simulink model "osek_led"  (Simulink 6.0)
settings: Solver=FixedStepDiscrete  StartTime=0.0  StopTime=100.0  RelTol=1e-3
undefined symbols (not defined in the file or in its folder): D4, D5, green, red
libraries: simulink x2, osekdrivers x2
settings Model: Creator=jcarrick  LastModifiedBy=jcarrick  ProdHWDeviceType=Motorola PowerPC
settings SolverCC: PositivePriorityOrder=on
settings DataIOCC: SaveOutput=off  SaveTime=off  SignalLoggingName=sigsOut
settings OptimizationCC: InlineInvariantSignals=off  OptimizeModelRefInitCode=on  LifeSpan=1
settings DebuggingCC: CheckExecutionContextPreStartOutputMsg=on  CheckExecutionContextRuntimeOutputMsg=on  SolverPrmCheckMsg=none
settings HardwareCC: ProdEndianess=BigEndian  ProdHWDeviceType=Motorola PowerPC
settings RTWCC: SystemTargetFile=osekworks.tlc  GenCodeOnly=on  TemplateMakefile=osek_default_tmf  GenerateReport=on  ProcessScript=osekworks_make_rtw_hook  IncludeHyperlinkInReport=on  LaunchReport=on
settings CodeAppCC: IgnoreCustomStorageClasses=off
settings STFCustomTargetCC: TargetFcnLib=ansi_tfl_tmw.mat  GenFloatMathFcnCalls=ANSI_C  ModelReferenceCompliant=off  CombineOutputUpdateFcns=on  SuppressErrorStatus=on  ERTCustomFileBanners=on  PurelyIntegerCode=on  SystemTargetFile=proosek.tlc  ForcedBaseTarget=off
settings ERTTargetCC: TargetFcnLib=ansi_tfl_tmw.mat  GenFloatMathFcnCalls=ANSI_C  ModelReferenceCompliant=off  SuppressErrorStatus=on  PurelyIntegerCode=on  SupportContinuousTime=on  SupportNonInlinedSFcns=on  RootIOFormat=Individual Arguments  ERTCustomFileTemplate=osek_file_process.tlc  InitialValueSource=Model
settings CustomProperty: DataType=RTWOptions_EnumType__toolbox_rtw_targets_osek_osek_osekworks_bspName  Value=phycore555
settings EnumStrPairs: String=axiomcmd565
settings SFSimCC: SFSimApplyToAllLibs=on  SFSimBuildMode=Incremental

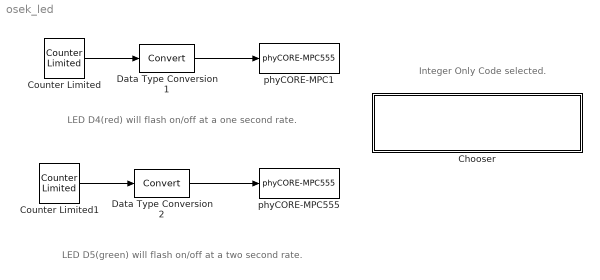
== system osek_led ==
  note: LED D4(red) will flash on/off at a one second rate.
  note: LED D5(green) will flash on/off at a two second rate.
  note: Integer Only Code selected.
  Chooser : Subsystem  LoadFcn=|  PropExecContextAcrossSSBoundary=on  mask{stf=osekworks.tlc}
      | x = osek.prefs.load('osek');                               
      | Implementation = lower(x.Implementation);                  
      | clear x;                                                   
      | switch Implementation                                      
      |  case {'proosek','osekworks'}                              
      |   osek_choose_imp([Implementation,'.tlc']);                
      |   set_param(gcb,'MaskValueString',[Implementation,'.tlc']);
      |  otherwise                                                 
      |   error(['Unrecognized implementation: ' Implementation]); 
      | end                                                        
      | clear Implementation;
      mask prompts: stf "Implementation"
      mask help: Choose OSEK System Target File
      mask init:
      | osek_choose_imp(stf)
      mask StyleString: popup(osekworks.tlc|proosek.tlc)
      mask Display: disp(['Choose System Target File:\nCurrently set to "' strtok(get_param(gcs,'rtwsystemtargetfile')) '"'])
  Counter Limited : simulink/Sources/Counter Limited  uplimit=1  tsamp=1
  Counter Limited1 : simulink/Sources/Counter Limited  uplimit=1  tsamp=2
  Data Type Conversion1 : DataTypeConversion  OutDataTypeMode=boolean  SaturateOnIntegerOverflow=on  RndMeth=Zero
  Data Type Conversion2 : DataTypeConversion  OutDataTypeMode=boolean  SaturateOnIntegerOverflow=on  RndMeth=Zero
  phyCORE-MPC1 : osekdrivers/phyCORE-MPC555  ledChoice=D4(red)
  phyCORE-MPC555 : osekdrivers/phyCORE-MPC555  ledChoice=D5(green)
  wires:
  Counter Limited/1 -> Data Type Conversion1/1
  Data Type Conversion1/1 -> phyCORE-MPC1/1
  Counter Limited1/1 -> Data Type Conversion2/1
  Data Type Conversion2/1 -> phyCORE-MPC555/1

== system osek_led/Chooser ==
